simulink model "Engine"  (R2024a)
settings: Solver=ode1be  StartTime=0.0  StopTime=10.0  FixedStep=0.001  RelTol=1e-3
undefined symbols (not defined in the file): cp, M_E, T_ini
settings Model: Creator=ojklem  LastModifiedBy=ojklem

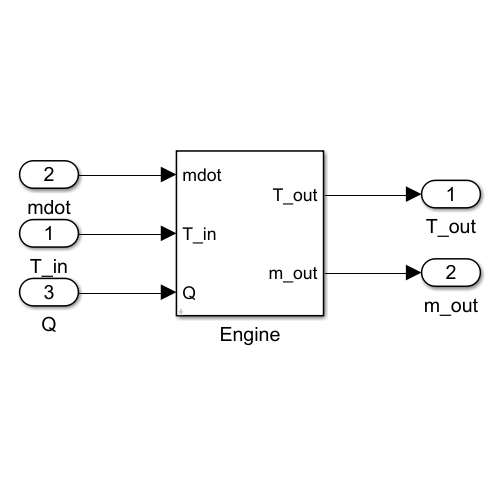
[thumbnail: Simulink's stored preview of the top-level diagram]
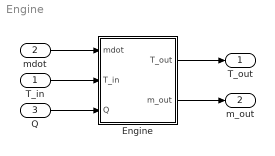
== system Engine ==
  T_in : Inport
  mdot : Inport  Port=2
  Q : Inport  Port=3
  Engine : Subsystem  mask{M=M_E, cp=cp}
      mask prompts: M "Mass [kg]"; cp "Specific heat capacity [J/kg/K]"
  T_out : Outport
  m_out : Outport  Port=2
  wires:
  T_in/1 -> Engine/2(T_in)
  mdot/1 -> Engine/1(mdot)
  Q/1 -> Engine/3(Q)
  Engine/1(T_out) -> T_out/1
  Engine/2(m_out) -> m_out/1

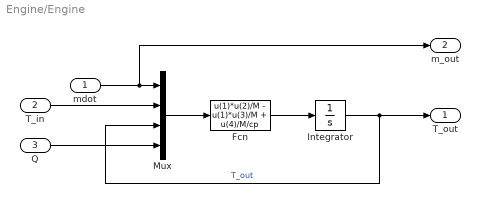
== system Engine/Engine ==
  mdot : Inport
  T_in : Inport  Port=2
  Q : Inport  Port=3
  Fcn : Fcn  Expr=u(1)*u(2)/M - u(1)*u(3)/M + u(4)/M/cp
  Integrator : Integrator  InitialCondition=T_ini
  Mux : Mux
  T_out : Outport
  m_out : Outport  Port=2
  wires:
  Integrator/1 -> Mux/3, T_out/1  "T_out"
  mdot/1 -> Mux/1, m_out/1
  Fcn/1 -> Integrator/1
  Mux/1 -> Fcn/1
  T_in/1 -> Mux/2
  Q/1 -> Mux/4
